simulink model "LyLStateCtrl"  (R2018b)
settings: Solver=FixedStepDiscrete  StartTime=0.0  StopTime=10.0  FixedStep=0.01  RelTol=1e-3
libraries: StateCtrlLib x1
settings Model: Creator=sn2xws  LastModifiedBy=sn2xws
settings DataIOCC: SaveFormat=StructureWithTime
settings OptimizationCC: DefaultParameterBehavior=Inlined  EnhancedBackFolding=on  PassReuseOutputArgsAs=Individual arguments  ZeroExternalMemoryAtStartup=off  ZeroInternalMemoryAtStartup=off  OptimizeBlockOrder=speed  DifferentSizesBufferReuse=on  OptimizationCustomize=off
settings DebuggingCC: ParameterTunabilityLossMsg=error
settings ModelReferenceCC: ModelReferenceNumInstancesAllowed=Single
settings SFSimCC: MATLABDynamicMemAlloc=off
settings RTWCC: SystemTargetFile=autosar.tlc  GenCodeOnly=on  TemplateMakefile=ert_default_tmf  Description=AUTOSAR  GenerateReport=on  IncludeHyperlinkInReport=on  LaunchReport=on  GenerateTraceInfo=on  GenerateTraceReport=on  GenerateTraceReportSl=on  GenerateTraceReportSf=on  GenerateTraceReportEml=on
settings CodeAppCC: ForceParamTrailComments=on  IgnoreCustomStorageClasses=off  OperatorAnnotations=on  SimulinkDataObjDesc=on  SFDataObjDesc=on  InsertBlockDesc=on
settings STFCustomTargetCC: TargetLangStandard=C99 (ISO)  MultiwordLength=256  ParMdlRefBuildCompliant=on  CompOptLevelCompliant=on  IncludeMdlTerminateFcn=off  CombineOutputUpdateFcns=on  SuppressErrorStatus=on  ERTCustomFileBanners=on  SupportNonFinite=off  SupportComplex=off  SupportContinuousTime=off  SupportNonInlinedSFcns=off  RemoveResetFunc=on  MATLABClassNameForMDSCustomization=Simulink.SoftwareTarget.ERTCustomization  AutosarCompliant=on  UseToolchainInfoCompliant=on  LookupTableObjectStructAxisOrder=2,1,3,4,...  LUTObjectStructOrderEvenSpacing=Size,Table,Breakpoints  SystemTargetFile=autosar.tlc
settings ERTTargetCC: TargetLangStandard=C99 (ISO)  ConcurrentExecutionCompliant=off  IncludeMdlTerminateFcn=off  SuppressErrorStatus=on  SupportNonFinite=off  SupportComplex=off  ModelStepFunctionPrototypeControlCompliant=off  CPPClassGenCompliant=off  AutosarCompliant=on  LookupTableObjectStructAxisOrder=2,1,3,4,...  LUTObjectStructOrderEvenSpacing=Size,Table,Breakpoints  InlinedParameterPlacement=NonHierarchical  ERTCustomFileTemplate=example_file_process.tlc

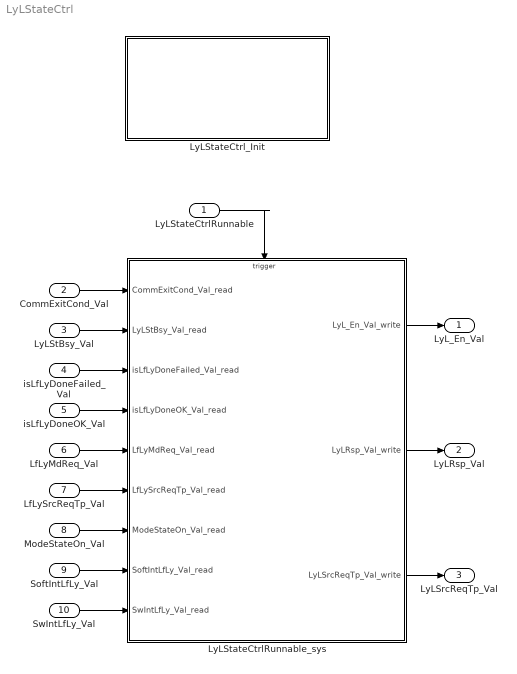
== system LyLStateCtrl ==
  LyLStateCtrlRunnable : Inport  SampleTime=0.01  OutputFunctionCall=on
  CommExitCond_Val : Inport  Port=2  OutDataTypeStr=boolean  PortDimensions=1
  LyLStBsy_Val : Inport  Port=3  OutDataTypeStr=boolean  PortDimensions=1
  isLfLyDoneFailed_Val : Inport  Port=4  OutDataTypeStr=boolean  PortDimensions=1
  isLfLyDoneOK_Val : Inport  Port=5  OutDataTypeStr=boolean  PortDimensions=1
  LfLyMdReq_Val : Inport  Port=6  OutDataTypeStr=boolean  PortDimensions=1
  LfLySrcReqTp_Val : Inport  Port=7  OutDataTypeStr=Enum: SrcReqTp1  PortDimensions=1
  ModeStateOn_Val : Inport  Port=8  OutDataTypeStr=boolean  PortDimensions=1
  SoftIntLfLy_Val : Inport  Port=9  OutDataTypeStr=IntEnable  PortDimensions=1
  SwIntLfLy_Val : Inport  Port=10  OutDataTypeStr=IntEnable  PortDimensions=1
  LyLStateCtrlRunnable_sys : Subsystem
  LyLStateCtrl_Init : Subsystem
  LyL_En_Val : Outport  OutDataTypeStr=boolean  PortDimensions=1
  LyLRsp_Val : Outport  Port=2  OutDataTypeStr=Enum: MdRspLocal1  PortDimensions=1
  LyLSrcReqTp_Val : Outport  Port=3  OutDataTypeStr=Enum: SrcReqTp1  PortDimensions=1
  wires:
  CommExitCond_Val/1 -> LyLStateCtrlRunnable_sys/1(CommExitCond_Val_read)
  LyLStBsy_Val/1 -> LyLStateCtrlRunnable_sys/2(LyLStBsy_Val_read)
  isLfLyDoneFailed_Val/1 -> LyLStateCtrlRunnable_sys/3(isLfLyDoneFailed_Val_read)
  isLfLyDoneOK_Val/1 -> LyLStateCtrlRunnable_sys/4(isLfLyDoneOK_Val_read)
  LfLyMdReq_Val/1 -> LyLStateCtrlRunnable_sys/5(LfLyMdReq_Val_read)
  LfLySrcReqTp_Val/1 -> LyLStateCtrlRunnable_sys/6(LfLySrcReqTp_Val_read)
  ModeStateOn_Val/1 -> LyLStateCtrlRunnable_sys/7(ModeStateOn_Val_read)
  SoftIntLfLy_Val/1 -> LyLStateCtrlRunnable_sys/8(SoftIntLfLy_Val_read)
  SwIntLfLy_Val/1 -> LyLStateCtrlRunnable_sys/9(SwIntLfLy_Val_read)
  LyLStateCtrlRunnable_sys/1(LyL_En_Val_write) -> LyL_En_Val/1
  LyLStateCtrlRunnable_sys/2(LyLRsp_Val_write) -> LyLRsp_Val/1
  LyLStateCtrlRunnable_sys/3(LyLSrcReqTp_Val_write) -> LyLSrcReqTp_Val/1
  LyLStateCtrlRunnable/1 -> LyLStateCtrlRunnable_sys/Trigger

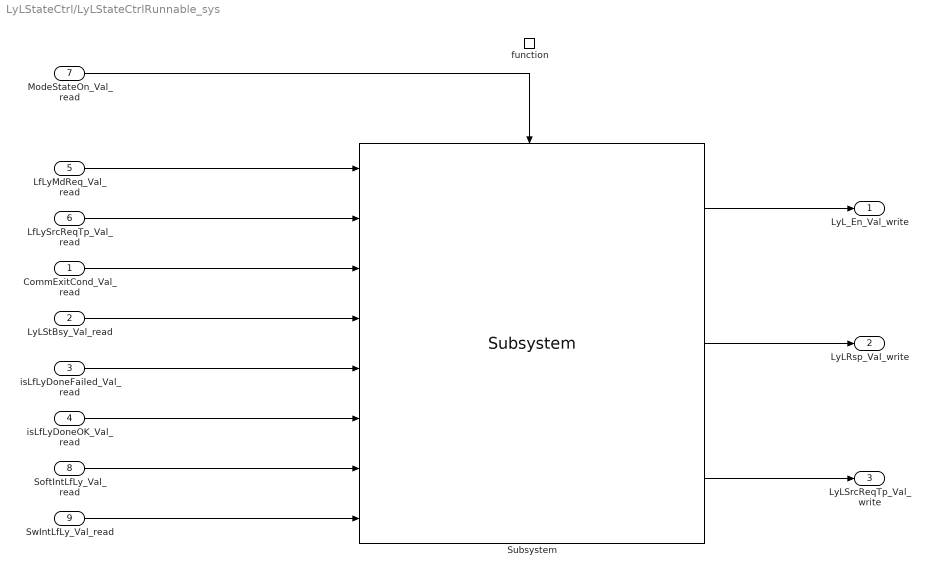
== system LyLStateCtrl/LyLStateCtrlRunnable_sys ==
  CommExitCond_Val_read : Inport
  LyLStBsy_Val_read : Inport  Port=2
  isLfLyDoneFailed_Val_read : Inport  Port=3
  isLfLyDoneOK_Val_read : Inport  Port=4
  LfLyMdReq_Val_read : Inport  Port=5
  LfLySrcReqTp_Val_read : Inport  Port=6
  ModeStateOn_Val_read : Inport  Port=7
  SoftIntLfLy_Val_read : Inport  Port=8  OutDataTypeStr=IntEnable
  SwIntLfLy_Val_read : Inport  Port=9  OutDataTypeStr=IntEnable
  function : TriggerPort  TriggerType=function-call  VariantControl=(inherit)  SampleTimeType=periodic  SampleTime=-1
  Subsystem : StateCtrlLib/Subsystem  SystemSampleTime=-1
  LyL_En_Val_write : Outport
      settings: EnsureOutportIsVirtual=on
  LyLRsp_Val_write : Outport  Port=2
      settings: EnsureOutportIsVirtual=on
  LyLSrcReqTp_Val_write : Outport  Port=3
      settings: EnsureOutportIsVirtual=on
  wires:
  LfLyMdReq_Val_read/1 -> Subsystem/1
  LfLySrcReqTp_Val_read/1 -> Subsystem/2
  isLfLyDoneOK_Val_read/1 -> Subsystem/6
  isLfLyDoneFailed_Val_read/1 -> Subsystem/5
  SoftIntLfLy_Val_read/1 -> Subsystem/7
  LyLStBsy_Val_read/1 -> Subsystem/4
  SwIntLfLy_Val_read/1 -> Subsystem/8
  CommExitCond_Val_read/1 -> Subsystem/3
  Subsystem/1 -> LyL_En_Val_write/1
  Subsystem/2 -> LyLRsp_Val_write/1
  Subsystem/3 -> LyLSrcReqTp_Val_write/1
  ModeStateOn_Val_read/1 -> Subsystem/Enable

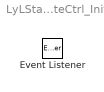
== system LyLStateCtrl/LyLStateCtrl_Init ==
  Event Listener : EventListener  EventName=reset
